simulink model "sim_M_test"  (R2015b)
settings: Solver=FixedStepAuto  StartTime=0.0  StopTime=10.0  RelTol=1e-3
libraries: simulink x3
settings Model: Creator=goat  LastModifiedBy=dell

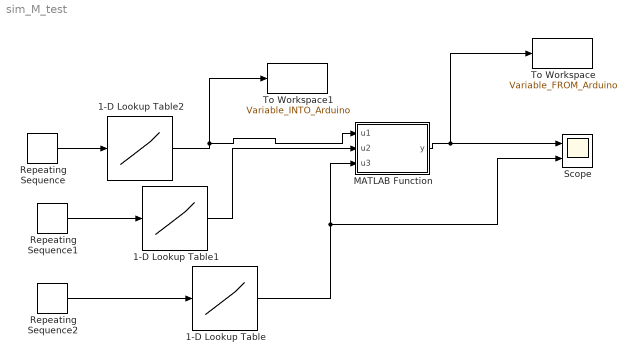
== system sim_M_test ==
  1-D Lookup Table : Lookup_n-D  NumberOfTableDimensions=1  BreakpointsForDimension1=[0:0.2:1.8]  Table=[ 1 2 3 4 5 6 7 8 9 10]  InternalRulePriority=Speed  RndMeth=Simplest  InputSameDT=on
  1-D Lookup Table1 : Lookup_n-D  NumberOfTableDimensions=1  BreakpointsForDimension1=[0:0.2:1.8]  Table=[ 1 2 3 4 5 6 7 8 9 10]  InternalRulePriority=Speed  RndMeth=Simplest  InputSameDT=on
  1-D Lookup Table2 : Lookup_n-D  NumberOfTableDimensions=1  BreakpointsForDimension1=[0:0.2:1.8]  Table=[ 1 2 3 4 5 6 7 8 9 10]  InternalRulePriority=Speed  RndMeth=Simplest  InputSameDT=on
  MATLAB Function : MATLAB Function  TreatAsAtomicUnit=on
  Repeating Sequence : simulink/Sources/Repeating Sequence  rep_seq_t=[0 2]  rep_seq_y=[0 2]
  Repeating Sequence1 : simulink/Sources/Repeating Sequence  rep_seq_t=[0 2]  rep_seq_y=[0 2]
  Repeating Sequence2 : simulink/Sources/Repeating Sequence  rep_seq_t=[0 2]  rep_seq_y=[0 2]
  Scope : Scope  NumInputPorts=2
  To Workspace : ToWorkspace  VariableName=Variable_FROM_Arduino  SaveFormat=Timeseries  SampleTime=-1
  To Workspace1 : ToWorkspace  VariableName=Variable_INTO_Arduino  SaveFormat=Timeseries  SampleTime=-1
  wires:
  Repeating Sequence/1 -> 1-D Lookup Table2/1
  MATLAB Function/1(y) -> To Workspace/1, Scope/1
  Repeating Sequence1/1 -> 1-D Lookup Table1/1
  Repeating Sequence2/1 -> 1-D Lookup Table/1
  1-D Lookup Table/1 -> Scope/2, MATLAB Function/3(u3)
  1-D Lookup Table1/1 -> MATLAB Function/2(u2)
  1-D Lookup Table2/1 -> To Workspace1/1, MATLAB Function/1(u1)

== matlab function sim_M_test/MATLAB Function ==
  data: u1 input; y output; u2 input; u3 input
function y = fcn(u1,u2,u3)
%#codegen
coder.extrinsic('mtlb_ardn_func','num2str') 
% u='1,2,32';
% u=[num2str(u1) ',' num2str(u2)  ',' num2str(u3) ];
y=1;%声明变量类型
y=mtlb_ardn_func([num2str(u1) ',' num2str(u2)  ',' num2str(u3) ])
